simulink model "fec_ber_hw"  (R2020b)
settings: Solver=FixedStepDiscrete  StartTime=0.0  StopTime=T/2  RelTol=1e-3
values from neighbouring files (symbols this model uses):
  aximm_awgn_reset = 0    [setup.m]
  aximm_bit_count_reset = 0    [setup.m]
  aximm_bits = n_blocks * k    (= 3200)    [setup.m]
  aximm_ctrl_word_dec = 0    [setup.m]
  aximm_ctrl_word_enc = 0    [setup.m]
  aximm_enable = 1    [setup.m]
  aximm_length = k * n_blocks    (= 3200)    [setup.m]
  aximm_length_dec = n    (= 160)    [setup.m]
  aximm_length_enc = k    (= 80)    [setup.m]
  aximm_llr_mag_reset = 0    [setup.m]
  aximm_llr_scale = (1/noise_var) * llr_scale    (= 1000)    [setup.m]
  aximm_load_dec = 1    [setup.m]
  aximm_load_enc = 1    [setup.m]
  aximm_noise_std = sqrt(noise_var)    [setup.m]
  aximm_reset = 0    [setup.m]
  d = sqrt(-2*log([0:1/4095:1]))    [setup.m]
  fs = 160e6    (= 160000000)    [setup.m]
  llr_scale = 7.75/7.75    (= 1)    [setup.m]
libraries: simulink x450, hdlsllib x190, commseqgen3 x20, dspsigops x17, lib_rfsoc_fec x5, commblkcod2 x3
(part 22 of 22)

== system fec_ber_hw/Soft Demodulation/SSR Soft Demodulation Lane 1/Soft Demodulation 7/Subsystem1/get_min1 ==
  a : Inport
  b : Inport  Port=2
  Compare To Zero : simulink/Logic and Bit Operations/Compare To Zero  relop=<=  OutDataTypeStr=boolean
  Multiport Switch2 : MultiPortSwitch  DataPortOrder=Zero-based contiguous  Inputs=2  zeroidx=on
  Subtract18 : Sum  Inputs=+-  OutDataTypeStr=fixdt(1,(w+1)*2+2,f*2)  SaturateOnIntegerOverflow=on
  min : Outport
  wires:
  Subtract18/1 -> Compare To Zero/1
  b/1 -> Subtract18/2, Multiport Switch2/2
  a/1 -> Multiport Switch2/3, Subtract18/1
  Multiport Switch2/1 -> min/1
  Compare To Zero/1 -> Multiport Switch2/1

== system fec_ber_hw/Soft Demodulation/SSR Soft Demodulation Lane 1/Soft Demodulation 7/Subsystem1/get_min2 ==
  a : Inport
  b : Inport  Port=2
  Compare To Zero : simulink/Logic and Bit Operations/Compare To Zero  relop=<=  OutDataTypeStr=boolean
  Multiport Switch2 : MultiPortSwitch  DataPortOrder=Zero-based contiguous  Inputs=2  zeroidx=on
  Subtract18 : Sum  Inputs=+-  OutDataTypeStr=fixdt(1,(w+1)*2+2,f*2)  SaturateOnIntegerOverflow=on
  min : Outport
  wires:
  Compare To Zero/1 -> Multiport Switch2/1
  Multiport Switch2/1 -> min/1
  a/1 -> Subtract18/1, Multiport Switch2/3
  b/1 -> Multiport Switch2/2, Subtract18/2
  Subtract18/1 -> Compare To Zero/1

== system fec_ber_hw/Soft Demodulation/SSR Soft Demodulation Lane 1/Soft Demodulation 7/Subsystem1/get_min3 ==
  a : Inport
  b : Inport  Port=2
  Compare To Zero : simulink/Logic and Bit Operations/Compare To Zero  relop=<=  OutDataTypeStr=boolean
  Multiport Switch2 : MultiPortSwitch  DataPortOrder=Zero-based contiguous  Inputs=2  zeroidx=on
  Subtract18 : Sum  Inputs=+-  OutDataTypeStr=fixdt(1,(w+1)*2+2,f*2)  SaturateOnIntegerOverflow=on
  min : Outport
  wires:
  Subtract18/1 -> Compare To Zero/1
  b/1 -> Subtract18/2, Multiport Switch2/2
  a/1 -> Multiport Switch2/3, Subtract18/1
  Multiport Switch2/1 -> min/1
  Compare To Zero/1 -> Multiport Switch2/1

== system fec_ber_hw/Soft Demodulation/SSR Soft Demodulation Lane 1/Soft Demodulation 7/Subsystem1/get_min4 ==
  a : Inport
  b : Inport  Port=2
  Compare To Zero : simulink/Logic and Bit Operations/Compare To Zero  relop=<=  OutDataTypeStr=boolean
  Multiport Switch2 : MultiPortSwitch  DataPortOrder=Zero-based contiguous  Inputs=2  zeroidx=on
  Subtract18 : Sum  Inputs=+-  OutDataTypeStr=fixdt(1,(w+1)*2+2,f*2)  SaturateOnIntegerOverflow=on
  min : Outport
  wires:
  Compare To Zero/1 -> Multiport Switch2/1
  Multiport Switch2/1 -> min/1
  a/1 -> Subtract18/1, Multiport Switch2/3
  b/1 -> Multiport Switch2/2, Subtract18/2
  Subtract18/1 -> Compare To Zero/1

== system fec_ber_hw/Soft Demodulation/SSR Soft Demodulation Lane 1/Soft Demodulation 7/Subsystem1/get_min5 ==
  a : Inport
  b : Inport  Port=2
  Compare To Zero : simulink/Logic and Bit Operations/Compare To Zero  relop=<=  OutDataTypeStr=boolean
  Multiport Switch2 : MultiPortSwitch  DataPortOrder=Zero-based contiguous  Inputs=2  zeroidx=on
  Subtract18 : Sum  Inputs=+-  OutDataTypeStr=fixdt(1,(w+1)*2+2,f*2)  SaturateOnIntegerOverflow=on
  min : Outport
  wires:
  Subtract18/1 -> Compare To Zero/1
  b/1 -> Subtract18/2, Multiport Switch2/2
  a/1 -> Multiport Switch2/3, Subtract18/1
  Multiport Switch2/1 -> min/1
  Compare To Zero/1 -> Multiport Switch2/1

== system fec_ber_hw/Soft Demodulation/SSR Soft Demodulation Lane 1/Soft Demodulation 7/Subsystem1/get_min6 ==
  a : Inport
  b : Inport  Port=2
  Compare To Zero : simulink/Logic and Bit Operations/Compare To Zero  relop=<=  OutDataTypeStr=boolean
  Multiport Switch2 : MultiPortSwitch  DataPortOrder=Zero-based contiguous  Inputs=2  zeroidx=on
  Subtract18 : Sum  Inputs=+-  OutDataTypeStr=fixdt(1,(w+1)*2+2,f*2)  SaturateOnIntegerOverflow=on
  min : Outport
  wires:
  Compare To Zero/1 -> Multiport Switch2/1
  Multiport Switch2/1 -> min/1
  a/1 -> Subtract18/1, Multiport Switch2/3
  b/1 -> Multiport Switch2/2, Subtract18/2
  Subtract18/1 -> Compare To Zero/1

== system fec_ber_hw/Soft Demodulation/SSR Soft Demodulation Lane 1/Soft Demodulation 7/Subsystem1/get_min7 ==
  a : Inport
  b : Inport  Port=2
  Compare To Zero : simulink/Logic and Bit Operations/Compare To Zero  relop=<=  OutDataTypeStr=boolean
  Multiport Switch2 : MultiPortSwitch  DataPortOrder=Zero-based contiguous  Inputs=2  zeroidx=on
  Subtract18 : Sum  Inputs=+-  OutDataTypeStr=fixdt(1,(w+1)*2+2,f*2)  SaturateOnIntegerOverflow=on
  min : Outport
  wires:
  Compare To Zero/1 -> Multiport Switch2/1
  Multiport Switch2/1 -> min/1
  a/1 -> Subtract18/1, Multiport Switch2/3
  b/1 -> Multiport Switch2/2, Subtract18/2
  Subtract18/1 -> Compare To Zero/1

== system fec_ber_hw/Soft Demodulation/SSR Soft Demodulation Lane 1/Soft Demodulation 7/Subsystem2/get_min1 ==
  a : Inport
  b : Inport  Port=2
  Compare To Zero : simulink/Logic and Bit Operations/Compare To Zero  relop=<=  OutDataTypeStr=boolean
  Multiport Switch2 : MultiPortSwitch  DataPortOrder=Zero-based contiguous  Inputs=2  zeroidx=on
  Subtract18 : Sum  Inputs=+-  OutDataTypeStr=fixdt(1,(w+1)*2+2,f*2)  SaturateOnIntegerOverflow=on
  min : Outport
  wires:
  Subtract18/1 -> Compare To Zero/1
  b/1 -> Subtract18/2, Multiport Switch2/2
  a/1 -> Multiport Switch2/3, Subtract18/1
  Multiport Switch2/1 -> min/1
  Compare To Zero/1 -> Multiport Switch2/1

== system fec_ber_hw/Soft Demodulation/SSR Soft Demodulation Lane 1/Soft Demodulation 7/Subsystem2/get_min2 ==
  a : Inport
  b : Inport  Port=2
  Compare To Zero : simulink/Logic and Bit Operations/Compare To Zero  relop=<=  OutDataTypeStr=boolean
  Multiport Switch2 : MultiPortSwitch  DataPortOrder=Zero-based contiguous  Inputs=2  zeroidx=on
  Subtract18 : Sum  Inputs=+-  OutDataTypeStr=fixdt(1,(w+1)*2+2,f*2)  SaturateOnIntegerOverflow=on
  min : Outport
  wires:
  Compare To Zero/1 -> Multiport Switch2/1
  Multiport Switch2/1 -> min/1
  a/1 -> Subtract18/1, Multiport Switch2/3
  b/1 -> Multiport Switch2/2, Subtract18/2
  Subtract18/1 -> Compare To Zero/1

== system fec_ber_hw/Soft Demodulation/SSR Soft Demodulation Lane 1/Soft Demodulation 7/Subsystem2/get_min3 ==
  a : Inport
  b : Inport  Port=2
  Compare To Zero : simulink/Logic and Bit Operations/Compare To Zero  relop=<=  OutDataTypeStr=boolean
  Multiport Switch2 : MultiPortSwitch  DataPortOrder=Zero-based contiguous  Inputs=2  zeroidx=on
  Subtract18 : Sum  Inputs=+-  OutDataTypeStr=fixdt(1,(w+1)*2+2,f*2)  SaturateOnIntegerOverflow=on
  min : Outport
  wires:
  Subtract18/1 -> Compare To Zero/1
  b/1 -> Subtract18/2, Multiport Switch2/2
  a/1 -> Multiport Switch2/3, Subtract18/1
  Multiport Switch2/1 -> min/1
  Compare To Zero/1 -> Multiport Switch2/1

== system fec_ber_hw/Soft Demodulation/SSR Soft Demodulation Lane 1/Soft Demodulation 7/Subsystem2/get_min4 ==
  a : Inport
  b : Inport  Port=2
  Compare To Zero : simulink/Logic and Bit Operations/Compare To Zero  relop=<=  OutDataTypeStr=boolean
  Multiport Switch2 : MultiPortSwitch  DataPortOrder=Zero-based contiguous  Inputs=2  zeroidx=on
  Subtract18 : Sum  Inputs=+-  OutDataTypeStr=fixdt(1,(w+1)*2+2,f*2)  SaturateOnIntegerOverflow=on
  min : Outport
  wires:
  Compare To Zero/1 -> Multiport Switch2/1
  Multiport Switch2/1 -> min/1
  a/1 -> Subtract18/1, Multiport Switch2/3
  b/1 -> Multiport Switch2/2, Subtract18/2
  Subtract18/1 -> Compare To Zero/1

== system fec_ber_hw/Soft Demodulation/SSR Soft Demodulation Lane 1/Soft Demodulation 7/Subsystem2/get_min5 ==
  a : Inport
  b : Inport  Port=2
  Compare To Zero : simulink/Logic and Bit Operations/Compare To Zero  relop=<=  OutDataTypeStr=boolean
  Multiport Switch2 : MultiPortSwitch  DataPortOrder=Zero-based contiguous  Inputs=2  zeroidx=on
  Subtract18 : Sum  Inputs=+-  OutDataTypeStr=fixdt(1,(w+1)*2+2,f*2)  SaturateOnIntegerOverflow=on
  min : Outport
  wires:
  Subtract18/1 -> Compare To Zero/1
  b/1 -> Subtract18/2, Multiport Switch2/2
  a/1 -> Multiport Switch2/3, Subtract18/1
  Multiport Switch2/1 -> min/1
  Compare To Zero/1 -> Multiport Switch2/1

== system fec_ber_hw/Soft Demodulation/SSR Soft Demodulation Lane 1/Soft Demodulation 7/Subsystem2/get_min6 ==
  a : Inport
  b : Inport  Port=2
  Compare To Zero : simulink/Logic and Bit Operations/Compare To Zero  relop=<=  OutDataTypeStr=boolean
  Multiport Switch2 : MultiPortSwitch  DataPortOrder=Zero-based contiguous  Inputs=2  zeroidx=on
  Subtract18 : Sum  Inputs=+-  OutDataTypeStr=fixdt(1,(w+1)*2+2,f*2)  SaturateOnIntegerOverflow=on
  min : Outport
  wires:
  Compare To Zero/1 -> Multiport Switch2/1
  Multiport Switch2/1 -> min/1
  a/1 -> Subtract18/1, Multiport Switch2/3
  b/1 -> Multiport Switch2/2, Subtract18/2
  Subtract18/1 -> Compare To Zero/1

== system fec_ber_hw/Soft Demodulation/SSR Soft Demodulation Lane 1/Soft Demodulation 7/Subsystem2/get_min7 ==
  a : Inport
  b : Inport  Port=2
  Compare To Zero : simulink/Logic and Bit Operations/Compare To Zero  relop=<=  OutDataTypeStr=boolean
  Multiport Switch2 : MultiPortSwitch  DataPortOrder=Zero-based contiguous  Inputs=2  zeroidx=on
  Subtract18 : Sum  Inputs=+-  OutDataTypeStr=fixdt(1,(w+1)*2+2,f*2)  SaturateOnIntegerOverflow=on
  min : Outport
  wires:
  Compare To Zero/1 -> Multiport Switch2/1
  Multiport Switch2/1 -> min/1
  a/1 -> Subtract18/1, Multiport Switch2/3
  b/1 -> Multiport Switch2/2, Subtract18/2
  Subtract18/1 -> Compare To Zero/1

== system fec_ber_hw/Soft Demodulation/SSR Soft Demodulation Lane 1/Soft Demodulation 8/Subsystem1/get_min1 ==
  a : Inport
  b : Inport  Port=2
  Compare To Zero : simulink/Logic and Bit Operations/Compare To Zero  relop=<=  OutDataTypeStr=boolean
  Multiport Switch2 : MultiPortSwitch  DataPortOrder=Zero-based contiguous  Inputs=2  zeroidx=on
  Subtract18 : Sum  Inputs=+-  OutDataTypeStr=fixdt(1,(w+1)*2+2,f*2)  SaturateOnIntegerOverflow=on
  min : Outport
  wires:
  Subtract18/1 -> Compare To Zero/1
  b/1 -> Subtract18/2, Multiport Switch2/2
  a/1 -> Multiport Switch2/3, Subtract18/1
  Multiport Switch2/1 -> min/1
  Compare To Zero/1 -> Multiport Switch2/1

== system fec_ber_hw/Soft Demodulation/SSR Soft Demodulation Lane 1/Soft Demodulation 8/Subsystem1/get_min2 ==
  a : Inport
  b : Inport  Port=2
  Compare To Zero : simulink/Logic and Bit Operations/Compare To Zero  relop=<=  OutDataTypeStr=boolean
  Multiport Switch2 : MultiPortSwitch  DataPortOrder=Zero-based contiguous  Inputs=2  zeroidx=on
  Subtract18 : Sum  Inputs=+-  OutDataTypeStr=fixdt(1,(w+1)*2+2,f*2)  SaturateOnIntegerOverflow=on
  min : Outport
  wires:
  Compare To Zero/1 -> Multiport Switch2/1
  Multiport Switch2/1 -> min/1
  a/1 -> Subtract18/1, Multiport Switch2/3
  b/1 -> Multiport Switch2/2, Subtract18/2
  Subtract18/1 -> Compare To Zero/1

== system fec_ber_hw/Soft Demodulation/SSR Soft Demodulation Lane 1/Soft Demodulation 8/Subsystem1/get_min3 ==
  a : Inport
  b : Inport  Port=2
  Compare To Zero : simulink/Logic and Bit Operations/Compare To Zero  relop=<=  OutDataTypeStr=boolean
  Multiport Switch2 : MultiPortSwitch  DataPortOrder=Zero-based contiguous  Inputs=2  zeroidx=on
  Subtract18 : Sum  Inputs=+-  OutDataTypeStr=fixdt(1,(w+1)*2+2,f*2)  SaturateOnIntegerOverflow=on
  min : Outport
  wires:
  Subtract18/1 -> Compare To Zero/1
  b/1 -> Subtract18/2, Multiport Switch2/2
  a/1 -> Multiport Switch2/3, Subtract18/1
  Multiport Switch2/1 -> min/1
  Compare To Zero/1 -> Multiport Switch2/1

== system fec_ber_hw/Soft Demodulation/SSR Soft Demodulation Lane 1/Soft Demodulation 8/Subsystem1/get_min4 ==
  a : Inport
  b : Inport  Port=2
  Compare To Zero : simulink/Logic and Bit Operations/Compare To Zero  relop=<=  OutDataTypeStr=boolean
  Multiport Switch2 : MultiPortSwitch  DataPortOrder=Zero-based contiguous  Inputs=2  zeroidx=on
  Subtract18 : Sum  Inputs=+-  OutDataTypeStr=fixdt(1,(w+1)*2+2,f*2)  SaturateOnIntegerOverflow=on
  min : Outport
  wires:
  Compare To Zero/1 -> Multiport Switch2/1
  Multiport Switch2/1 -> min/1
  a/1 -> Subtract18/1, Multiport Switch2/3
  b/1 -> Multiport Switch2/2, Subtract18/2
  Subtract18/1 -> Compare To Zero/1

== system fec_ber_hw/Soft Demodulation/SSR Soft Demodulation Lane 1/Soft Demodulation 8/Subsystem1/get_min5 ==
  a : Inport
  b : Inport  Port=2
  Compare To Zero : simulink/Logic and Bit Operations/Compare To Zero  relop=<=  OutDataTypeStr=boolean
  Multiport Switch2 : MultiPortSwitch  DataPortOrder=Zero-based contiguous  Inputs=2  zeroidx=on
  Subtract18 : Sum  Inputs=+-  OutDataTypeStr=fixdt(1,(w+1)*2+2,f*2)  SaturateOnIntegerOverflow=on
  min : Outport
  wires:
  Subtract18/1 -> Compare To Zero/1
  b/1 -> Subtract18/2, Multiport Switch2/2
  a/1 -> Multiport Switch2/3, Subtract18/1
  Multiport Switch2/1 -> min/1
  Compare To Zero/1 -> Multiport Switch2/1

== system fec_ber_hw/Soft Demodulation/SSR Soft Demodulation Lane 1/Soft Demodulation 8/Subsystem1/get_min6 ==
  a : Inport
  b : Inport  Port=2
  Compare To Zero : simulink/Logic and Bit Operations/Compare To Zero  relop=<=  OutDataTypeStr=boolean
  Multiport Switch2 : MultiPortSwitch  DataPortOrder=Zero-based contiguous  Inputs=2  zeroidx=on
  Subtract18 : Sum  Inputs=+-  OutDataTypeStr=fixdt(1,(w+1)*2+2,f*2)  SaturateOnIntegerOverflow=on
  min : Outport
  wires:
  Compare To Zero/1 -> Multiport Switch2/1
  Multiport Switch2/1 -> min/1
  a/1 -> Subtract18/1, Multiport Switch2/3
  b/1 -> Multiport Switch2/2, Subtract18/2
  Subtract18/1 -> Compare To Zero/1

== system fec_ber_hw/Soft Demodulation/SSR Soft Demodulation Lane 1/Soft Demodulation 8/Subsystem1/get_min7 ==
  a : Inport
  b : Inport  Port=2
  Compare To Zero : simulink/Logic and Bit Operations/Compare To Zero  relop=<=  OutDataTypeStr=boolean
  Multiport Switch2 : MultiPortSwitch  DataPortOrder=Zero-based contiguous  Inputs=2  zeroidx=on
  Subtract18 : Sum  Inputs=+-  OutDataTypeStr=fixdt(1,(w+1)*2+2,f*2)  SaturateOnIntegerOverflow=on
  min : Outport
  wires:
  Compare To Zero/1 -> Multiport Switch2/1
  Multiport Switch2/1 -> min/1
  a/1 -> Subtract18/1, Multiport Switch2/3
  b/1 -> Multiport Switch2/2, Subtract18/2
  Subtract18/1 -> Compare To Zero/1

== system fec_ber_hw/Soft Demodulation/SSR Soft Demodulation Lane 1/Soft Demodulation 8/Subsystem2/get_min1 ==
  a : Inport
  b : Inport  Port=2
  Compare To Zero : simulink/Logic and Bit Operations/Compare To Zero  relop=<=  OutDataTypeStr=boolean
  Multiport Switch2 : MultiPortSwitch  DataPortOrder=Zero-based contiguous  Inputs=2  zeroidx=on
  Subtract18 : Sum  Inputs=+-  OutDataTypeStr=fixdt(1,(w+1)*2+2,f*2)  SaturateOnIntegerOverflow=on
  min : Outport
  wires:
  Subtract18/1 -> Compare To Zero/1
  b/1 -> Subtract18/2, Multiport Switch2/2
  a/1 -> Multiport Switch2/3, Subtract18/1
  Multiport Switch2/1 -> min/1
  Compare To Zero/1 -> Multiport Switch2/1

== system fec_ber_hw/Soft Demodulation/SSR Soft Demodulation Lane 1/Soft Demodulation 8/Subsystem2/get_min2 ==
  a : Inport
  b : Inport  Port=2
  Compare To Zero : simulink/Logic and Bit Operations/Compare To Zero  relop=<=  OutDataTypeStr=boolean
  Multiport Switch2 : MultiPortSwitch  DataPortOrder=Zero-based contiguous  Inputs=2  zeroidx=on
  Subtract18 : Sum  Inputs=+-  OutDataTypeStr=fixdt(1,(w+1)*2+2,f*2)  SaturateOnIntegerOverflow=on
  min : Outport
  wires:
  Compare To Zero/1 -> Multiport Switch2/1
  Multiport Switch2/1 -> min/1
  a/1 -> Subtract18/1, Multiport Switch2/3
  b/1 -> Multiport Switch2/2, Subtract18/2
  Subtract18/1 -> Compare To Zero/1

== system fec_ber_hw/Soft Demodulation/SSR Soft Demodulation Lane 1/Soft Demodulation 8/Subsystem2/get_min3 ==
  a : Inport
  b : Inport  Port=2
  Compare To Zero : simulink/Logic and Bit Operations/Compare To Zero  relop=<=  OutDataTypeStr=boolean
  Multiport Switch2 : MultiPortSwitch  DataPortOrder=Zero-based contiguous  Inputs=2  zeroidx=on
  Subtract18 : Sum  Inputs=+-  OutDataTypeStr=fixdt(1,(w+1)*2+2,f*2)  SaturateOnIntegerOverflow=on
  min : Outport
  wires:
  Subtract18/1 -> Compare To Zero/1
  b/1 -> Subtract18/2, Multiport Switch2/2
  a/1 -> Multiport Switch2/3, Subtract18/1
  Multiport Switch2/1 -> min/1
  Compare To Zero/1 -> Multiport Switch2/1

== system fec_ber_hw/Soft Demodulation/SSR Soft Demodulation Lane 1/Soft Demodulation 8/Subsystem2/get_min4 ==
  a : Inport
  b : Inport  Port=2
  Compare To Zero : simulink/Logic and Bit Operations/Compare To Zero  relop=<=  OutDataTypeStr=boolean
  Multiport Switch2 : MultiPortSwitch  DataPortOrder=Zero-based contiguous  Inputs=2  zeroidx=on
  Subtract18 : Sum  Inputs=+-  OutDataTypeStr=fixdt(1,(w+1)*2+2,f*2)  SaturateOnIntegerOverflow=on
  min : Outport
  wires:
  Compare To Zero/1 -> Multiport Switch2/1
  Multiport Switch2/1 -> min/1
  a/1 -> Subtract18/1, Multiport Switch2/3
  b/1 -> Multiport Switch2/2, Subtract18/2
  Subtract18/1 -> Compare To Zero/1

== system fec_ber_hw/Soft Demodulation/SSR Soft Demodulation Lane 1/Soft Demodulation 8/Subsystem2/get_min5 ==
  a : Inport
  b : Inport  Port=2
  Compare To Zero : simulink/Logic and Bit Operations/Compare To Zero  relop=<=  OutDataTypeStr=boolean
  Multiport Switch2 : MultiPortSwitch  DataPortOrder=Zero-based contiguous  Inputs=2  zeroidx=on
  Subtract18 : Sum  Inputs=+-  OutDataTypeStr=fixdt(1,(w+1)*2+2,f*2)  SaturateOnIntegerOverflow=on
  min : Outport
  wires:
  Subtract18/1 -> Compare To Zero/1
  b/1 -> Subtract18/2, Multiport Switch2/2
  a/1 -> Multiport Switch2/3, Subtract18/1
  Multiport Switch2/1 -> min/1
  Compare To Zero/1 -> Multiport Switch2/1

== system fec_ber_hw/Soft Demodulation/SSR Soft Demodulation Lane 1/Soft Demodulation 8/Subsystem2/get_min6 ==
  a : Inport
  b : Inport  Port=2
  Compare To Zero : simulink/Logic and Bit Operations/Compare To Zero  relop=<=  OutDataTypeStr=boolean
  Multiport Switch2 : MultiPortSwitch  DataPortOrder=Zero-based contiguous  Inputs=2  zeroidx=on
  Subtract18 : Sum  Inputs=+-  OutDataTypeStr=fixdt(1,(w+1)*2+2,f*2)  SaturateOnIntegerOverflow=on
  min : Outport
  wires:
  Compare To Zero/1 -> Multiport Switch2/1
  Multiport Switch2/1 -> min/1
  a/1 -> Subtract18/1, Multiport Switch2/3
  b/1 -> Multiport Switch2/2, Subtract18/2
  Subtract18/1 -> Compare To Zero/1

== system fec_ber_hw/Soft Demodulation/SSR Soft Demodulation Lane 1/Soft Demodulation 8/Subsystem2/get_min7 ==
  a : Inport
  b : Inport  Port=2
  Compare To Zero : simulink/Logic and Bit Operations/Compare To Zero  relop=<=  OutDataTypeStr=boolean
  Multiport Switch2 : MultiPortSwitch  DataPortOrder=Zero-based contiguous  Inputs=2  zeroidx=on
  Subtract18 : Sum  Inputs=+-  OutDataTypeStr=fixdt(1,(w+1)*2+2,f*2)  SaturateOnIntegerOverflow=on
  min : Outport
  wires:
  Compare To Zero/1 -> Multiport Switch2/1
  Multiport Switch2/1 -> min/1
  a/1 -> Subtract18/1, Multiport Switch2/3
  b/1 -> Multiport Switch2/2, Subtract18/2
  Subtract18/1 -> Compare To Zero/1

== system fec_ber_hw/Soft Demodulation/SSR Soft Demodulation Lane 1/Soft Demodulation 9/Subsystem1/get_min1 ==
  a : Inport
  b : Inport  Port=2
  Compare To Zero : simulink/Logic and Bit Operations/Compare To Zero  relop=<=  OutDataTypeStr=boolean
  Multiport Switch2 : MultiPortSwitch  DataPortOrder=Zero-based contiguous  Inputs=2  zeroidx=on
  Subtract18 : Sum  Inputs=+-  OutDataTypeStr=fixdt(1,(w+1)*2+2,f*2)  SaturateOnIntegerOverflow=on
  min : Outport
  wires:
  Subtract18/1 -> Compare To Zero/1
  b/1 -> Subtract18/2, Multiport Switch2/2
  a/1 -> Multiport Switch2/3, Subtract18/1
  Multiport Switch2/1 -> min/1
  Compare To Zero/1 -> Multiport Switch2/1

== system fec_ber_hw/Soft Demodulation/SSR Soft Demodulation Lane 1/Soft Demodulation 9/Subsystem1/get_min2 ==
  a : Inport
  b : Inport  Port=2
  Compare To Zero : simulink/Logic and Bit Operations/Compare To Zero  relop=<=  OutDataTypeStr=boolean
  Multiport Switch2 : MultiPortSwitch  DataPortOrder=Zero-based contiguous  Inputs=2  zeroidx=on
  Subtract18 : Sum  Inputs=+-  OutDataTypeStr=fixdt(1,(w+1)*2+2,f*2)  SaturateOnIntegerOverflow=on
  min : Outport
  wires:
  Compare To Zero/1 -> Multiport Switch2/1
  Multiport Switch2/1 -> min/1
  a/1 -> Subtract18/1, Multiport Switch2/3
  b/1 -> Multiport Switch2/2, Subtract18/2
  Subtract18/1 -> Compare To Zero/1

== system fec_ber_hw/Soft Demodulation/SSR Soft Demodulation Lane 1/Soft Demodulation 9/Subsystem1/get_min3 ==
  a : Inport
  b : Inport  Port=2
  Compare To Zero : simulink/Logic and Bit Operations/Compare To Zero  relop=<=  OutDataTypeStr=boolean
  Multiport Switch2 : MultiPortSwitch  DataPortOrder=Zero-based contiguous  Inputs=2  zeroidx=on
  Subtract18 : Sum  Inputs=+-  OutDataTypeStr=fixdt(1,(w+1)*2+2,f*2)  SaturateOnIntegerOverflow=on
  min : Outport
  wires:
  Subtract18/1 -> Compare To Zero/1
  b/1 -> Subtract18/2, Multiport Switch2/2
  a/1 -> Multiport Switch2/3, Subtract18/1
  Multiport Switch2/1 -> min/1
  Compare To Zero/1 -> Multiport Switch2/1

== system fec_ber_hw/Soft Demodulation/SSR Soft Demodulation Lane 1/Soft Demodulation 9/Subsystem1/get_min4 ==
  a : Inport
  b : Inport  Port=2
  Compare To Zero : simulink/Logic and Bit Operations/Compare To Zero  relop=<=  OutDataTypeStr=boolean
  Multiport Switch2 : MultiPortSwitch  DataPortOrder=Zero-based contiguous  Inputs=2  zeroidx=on
  Subtract18 : Sum  Inputs=+-  OutDataTypeStr=fixdt(1,(w+1)*2+2,f*2)  SaturateOnIntegerOverflow=on
  min : Outport
  wires:
  Compare To Zero/1 -> Multiport Switch2/1
  Multiport Switch2/1 -> min/1
  a/1 -> Subtract18/1, Multiport Switch2/3
  b/1 -> Multiport Switch2/2, Subtract18/2
  Subtract18/1 -> Compare To Zero/1

== system fec_ber_hw/Soft Demodulation/SSR Soft Demodulation Lane 1/Soft Demodulation 9/Subsystem1/get_min5 ==
  a : Inport
  b : Inport  Port=2
  Compare To Zero : simulink/Logic and Bit Operations/Compare To Zero  relop=<=  OutDataTypeStr=boolean
  Multiport Switch2 : MultiPortSwitch  DataPortOrder=Zero-based contiguous  Inputs=2  zeroidx=on
  Subtract18 : Sum  Inputs=+-  OutDataTypeStr=fixdt(1,(w+1)*2+2,f*2)  SaturateOnIntegerOverflow=on
  min : Outport
  wires:
  Subtract18/1 -> Compare To Zero/1
  b/1 -> Subtract18/2, Multiport Switch2/2
  a/1 -> Multiport Switch2/3, Subtract18/1
  Multiport Switch2/1 -> min/1
  Compare To Zero/1 -> Multiport Switch2/1

== system fec_ber_hw/Soft Demodulation/SSR Soft Demodulation Lane 1/Soft Demodulation 9/Subsystem1/get_min6 ==
  a : Inport
  b : Inport  Port=2
  Compare To Zero : simulink/Logic and Bit Operations/Compare To Zero  relop=<=  OutDataTypeStr=boolean
  Multiport Switch2 : MultiPortSwitch  DataPortOrder=Zero-based contiguous  Inputs=2  zeroidx=on
  Subtract18 : Sum  Inputs=+-  OutDataTypeStr=fixdt(1,(w+1)*2+2,f*2)  SaturateOnIntegerOverflow=on
  min : Outport
  wires:
  Compare To Zero/1 -> Multiport Switch2/1
  Multiport Switch2/1 -> min/1
  a/1 -> Subtract18/1, Multiport Switch2/3
  b/1 -> Multiport Switch2/2, Subtract18/2
  Subtract18/1 -> Compare To Zero/1

== system fec_ber_hw/Soft Demodulation/SSR Soft Demodulation Lane 1/Soft Demodulation 9/Subsystem1/get_min7 ==
  a : Inport
  b : Inport  Port=2
  Compare To Zero : simulink/Logic and Bit Operations/Compare To Zero  relop=<=  OutDataTypeStr=boolean
  Multiport Switch2 : MultiPortSwitch  DataPortOrder=Zero-based contiguous  Inputs=2  zeroidx=on
  Subtract18 : Sum  Inputs=+-  OutDataTypeStr=fixdt(1,(w+1)*2+2,f*2)  SaturateOnIntegerOverflow=on
  min : Outport
  wires:
  Compare To Zero/1 -> Multiport Switch2/1
  Multiport Switch2/1 -> min/1
  a/1 -> Subtract18/1, Multiport Switch2/3
  b/1 -> Multiport Switch2/2, Subtract18/2
  Subtract18/1 -> Compare To Zero/1

== system fec_ber_hw/Soft Demodulation/SSR Soft Demodulation Lane 1/Soft Demodulation 9/Subsystem2/get_min1 ==
  a : Inport
  b : Inport  Port=2
  Compare To Zero : simulink/Logic and Bit Operations/Compare To Zero  relop=<=  OutDataTypeStr=boolean
  Multiport Switch2 : MultiPortSwitch  DataPortOrder=Zero-based contiguous  Inputs=2  zeroidx=on
  Subtract18 : Sum  Inputs=+-  OutDataTypeStr=fixdt(1,(w+1)*2+2,f*2)  SaturateOnIntegerOverflow=on
  min : Outport
  wires:
  Subtract18/1 -> Compare To Zero/1
  b/1 -> Subtract18/2, Multiport Switch2/2
  a/1 -> Multiport Switch2/3, Subtract18/1
  Multiport Switch2/1 -> min/1
  Compare To Zero/1 -> Multiport Switch2/1

== system fec_ber_hw/Soft Demodulation/SSR Soft Demodulation Lane 1/Soft Demodulation 9/Subsystem2/get_min2 ==
  a : Inport
  b : Inport  Port=2
  Compare To Zero : simulink/Logic and Bit Operations/Compare To Zero  relop=<=  OutDataTypeStr=boolean
  Multiport Switch2 : MultiPortSwitch  DataPortOrder=Zero-based contiguous  Inputs=2  zeroidx=on
  Subtract18 : Sum  Inputs=+-  OutDataTypeStr=fixdt(1,(w+1)*2+2,f*2)  SaturateOnIntegerOverflow=on
  min : Outport
  wires:
  Compare To Zero/1 -> Multiport Switch2/1
  Multiport Switch2/1 -> min/1
  a/1 -> Subtract18/1, Multiport Switch2/3
  b/1 -> Multiport Switch2/2, Subtract18/2
  Subtract18/1 -> Compare To Zero/1

== system fec_ber_hw/Soft Demodulation/SSR Soft Demodulation Lane 1/Soft Demodulation 9/Subsystem2/get_min3 ==
  a : Inport
  b : Inport  Port=2
  Compare To Zero : simulink/Logic and Bit Operations/Compare To Zero  relop=<=  OutDataTypeStr=boolean
  Multiport Switch2 : MultiPortSwitch  DataPortOrder=Zero-based contiguous  Inputs=2  zeroidx=on
  Subtract18 : Sum  Inputs=+-  OutDataTypeStr=fixdt(1,(w+1)*2+2,f*2)  SaturateOnIntegerOverflow=on
  min : Outport
  wires:
  Subtract18/1 -> Compare To Zero/1
  b/1 -> Subtract18/2, Multiport Switch2/2
  a/1 -> Multiport Switch2/3, Subtract18/1
  Multiport Switch2/1 -> min/1
  Compare To Zero/1 -> Multiport Switch2/1

== system fec_ber_hw/Soft Demodulation/SSR Soft Demodulation Lane 1/Soft Demodulation 9/Subsystem2/get_min4 ==
  a : Inport
  b : Inport  Port=2
  Compare To Zero : simulink/Logic and Bit Operations/Compare To Zero  relop=<=  OutDataTypeStr=boolean
  Multiport Switch2 : MultiPortSwitch  DataPortOrder=Zero-based contiguous  Inputs=2  zeroidx=on
  Subtract18 : Sum  Inputs=+-  OutDataTypeStr=fixdt(1,(w+1)*2+2,f*2)  SaturateOnIntegerOverflow=on
  min : Outport
  wires:
  Compare To Zero/1 -> Multiport Switch2/1
  Multiport Switch2/1 -> min/1
  a/1 -> Subtract18/1, Multiport Switch2/3
  b/1 -> Multiport Switch2/2, Subtract18/2
  Subtract18/1 -> Compare To Zero/1

== system fec_ber_hw/Soft Demodulation/SSR Soft Demodulation Lane 1/Soft Demodulation 9/Subsystem2/get_min5 ==
  a : Inport
  b : Inport  Port=2
  Compare To Zero : simulink/Logic and Bit Operations/Compare To Zero  relop=<=  OutDataTypeStr=boolean
  Multiport Switch2 : MultiPortSwitch  DataPortOrder=Zero-based contiguous  Inputs=2  zeroidx=on
  Subtract18 : Sum  Inputs=+-  OutDataTypeStr=fixdt(1,(w+1)*2+2,f*2)  SaturateOnIntegerOverflow=on
  min : Outport
  wires:
  Subtract18/1 -> Compare To Zero/1
  b/1 -> Subtract18/2, Multiport Switch2/2
  a/1 -> Multiport Switch2/3, Subtract18/1
  Multiport Switch2/1 -> min/1
  Compare To Zero/1 -> Multiport Switch2/1

== system fec_ber_hw/Soft Demodulation/SSR Soft Demodulation Lane 1/Soft Demodulation 9/Subsystem2/get_min6 ==
  a : Inport
  b : Inport  Port=2
  Compare To Zero : simulink/Logic and Bit Operations/Compare To Zero  relop=<=  OutDataTypeStr=boolean
  Multiport Switch2 : MultiPortSwitch  DataPortOrder=Zero-based contiguous  Inputs=2  zeroidx=on
  Subtract18 : Sum  Inputs=+-  OutDataTypeStr=fixdt(1,(w+1)*2+2,f*2)  SaturateOnIntegerOverflow=on
  min : Outport
  wires:
  Compare To Zero/1 -> Multiport Switch2/1
  Multiport Switch2/1 -> min/1
  a/1 -> Subtract18/1, Multiport Switch2/3
  b/1 -> Multiport Switch2/2, Subtract18/2
  Subtract18/1 -> Compare To Zero/1

== system fec_ber_hw/Soft Demodulation/SSR Soft Demodulation Lane 1/Soft Demodulation 9/Subsystem2/get_min7 ==
  a : Inport
  b : Inport  Port=2
  Compare To Zero : simulink/Logic and Bit Operations/Compare To Zero  relop=<=  OutDataTypeStr=boolean
  Multiport Switch2 : MultiPortSwitch  DataPortOrder=Zero-based contiguous  Inputs=2  zeroidx=on
  Subtract18 : Sum  Inputs=+-  OutDataTypeStr=fixdt(1,(w+1)*2+2,f*2)  SaturateOnIntegerOverflow=on
  min : Outport
  wires:
  Compare To Zero/1 -> Multiport Switch2/1
  Multiport Switch2/1 -> min/1
  a/1 -> Subtract18/1, Multiport Switch2/3
  b/1 -> Multiport Switch2/2, Subtract18/2
  Subtract18/1 -> Compare To Zero/1

== matlab function fec_ber_hw/Decode/MATLAB Function1 ==
  data: valid input; frame input; uint8 output [0..80]; k parameter
function uint8 = fcn(valid, frame, k)

persistent f u count

if isempty(f)
    f = zeros(1,8);
    u = fi(0,0,8,0);
    count = 0;
end

if valid
    f = frame((1:8)+(8*count));
    u(:) = f(8)*2^7 ...
      + f(7)*2^6 ...
      + f(6)*2^5 ...
      + f(5)*2^4 ...
      + f(4)*2^3 ...
      + f(3)*2^2 ...
      + f(2)*2^1 ...
      + f(1)*2^0;
  count = count + 1;
end

if count >= 10
    count = 0;
end

uint8 = u;

== matlab function fec_ber_hw/Soft Demodulation/SSR Soft Demodulation Lane 0/Soft Demodulation 2/symmetric_saturation ==
  data: u input; y output
function y = symmetric_saturation(u)
    if u > 7.75
        y = fi(7.75, 1, 6, 2);
    elseif u < -7.75
        y = fi(-7.75, 1, 6, 2);
    else
        y = fi(u, 1, 6, 2);
    end

== matlab function fec_ber_hw/Soft Demodulation/SSR Soft Demodulation Lane 0/Soft Demodulation 3/symmetric_saturation ==
  data: u input; y output
function y = symmetric_saturation(u)
    if u > 7.75
        y = fi(7.75, 1, 6, 2);
    elseif u < -7.75
        y = fi(-7.75, 1, 6, 2);
    else
        y = fi(u, 1, 6, 2);
    end

== matlab function fec_ber_hw/Soft Demodulation/SSR Soft Demodulation Lane 0/Soft Demodulation 4/symmetric_saturation ==
  data: u input; y output
function y = symmetric_saturation(u)
    if u > 7.75
        y = fi(7.75, 1, 6, 2);
    elseif u < -7.75
        y = fi(-7.75, 1, 6, 2);
    else
        y = fi(u, 1, 6, 2);
    end

== matlab function fec_ber_hw/Soft Demodulation/SSR Soft Demodulation Lane 0/Soft Demodulation 5/symmetric_saturation ==
  data: u input; y output
function y = symmetric_saturation(u)
    if u > 7.75
        y = fi(7.75, 1, 6, 2);
    elseif u < -7.75
        y = fi(-7.75, 1, 6, 2);
    else
        y = fi(u, 1, 6, 2);
    end

== matlab function fec_ber_hw/Soft Demodulation/SSR Soft Demodulation Lane 0/Soft Demodulation 6/symmetric_saturation ==
  data: u input; y output
function y = symmetric_saturation(u)
    if u > 7.75
        y = fi(7.75, 1, 6, 2);
    elseif u < -7.75
        y = fi(-7.75, 1, 6, 2);
    else
        y = fi(u, 1, 6, 2);
    end

== matlab function fec_ber_hw/Soft Demodulation/SSR Soft Demodulation Lane 0/Soft Demodulation 7/symmetric_saturation ==
  data: u input; y output
function y = symmetric_saturation(u)
    if u > 7.75
        y = fi(7.75, 1, 6, 2);
    elseif u < -7.75
        y = fi(-7.75, 1, 6, 2);
    else
        y = fi(u, 1, 6, 2);
    end

== matlab function fec_ber_hw/Soft Demodulation/SSR Soft Demodulation Lane 0/Soft Demodulation 8/symmetric_saturation ==
  data: u input; y output
function y = symmetric_saturation(u)
    if u > 7.75
        y = fi(7.75, 1, 6, 2);
    elseif u < -7.75
        y = fi(-7.75, 1, 6, 2);
    else
        y = fi(u, 1, 6, 2);
    end

== matlab function fec_ber_hw/Soft Demodulation/SSR Soft Demodulation Lane 0/Soft Demodulation 9/symmetric_saturation ==
  data: u input; y output
function y = symmetric_saturation(u)
    if u > 7.75
        y = fi(7.75, 1, 6, 2);
    elseif u < -7.75
        y = fi(-7.75, 1, 6, 2);
    else
        y = fi(u, 1, 6, 2);
    end

== matlab function fec_ber_hw/Soft Demodulation/SSR Soft Demodulation Lane 0/Soft Demodulation 10/symmetric_saturation ==
  data: u input; y output
function y = symmetric_saturation(u)
    if u > 7.75
        y = fi(7.75, 1, 6, 2);
    elseif u < -7.75
        y = fi(-7.75, 1, 6, 2);
    else
        y = fi(u, 1, 6, 2);
    end

== matlab function fec_ber_hw/Soft Demodulation/SSR Soft Demodulation Lane 0/Soft Demodulation 11/symmetric_saturation ==
  data: u input; y output
function y = symmetric_saturation(u)
    if u > 7.75
        y = fi(7.75, 1, 6, 2);
    elseif u < -7.75
        y = fi(-7.75, 1, 6, 2);
    else
        y = fi(u, 1, 6, 2);
    end

== matlab function fec_ber_hw/Soft Demodulation/SSR Soft Demodulation Lane 0/Soft Demodulation 12/symmetric_saturation ==
  data: u input; y output
function y = symmetric_saturation(u)
    if u > 7.75
        y = fi(7.75, 1, 6, 2);
    elseif u < -7.75
        y = fi(-7.75, 1, 6, 2);
    else
        y = fi(u, 1, 6, 2);
    end

== matlab function fec_ber_hw/Encoder/MATLAB Function4 ==
  data: bits input; valid input; frame input size=[160, 1]; tvalid output; lane_0 output size=[1,1]; lane_1 output size=[1,1]; lane_2 output size=[1,1]; lane_3 output; lane_4 output; lane_5 output; lane_6 output; lane_7 output
function [tvalid,lane_0,lane_1,lane_2,lane_3,lane_4,lane_5,lane_6,lane_7] = fcn(bits, valid, frame)

persistent n buffer w buf_i prev_buffer b empty_flag clock_count

if isempty(n)
    n = 160;
    w = 64;
    b = 0;
    prev_buffer = false(1,w*8*4)';
    buffer = false(1,w*8*4)';
    buf_i = 1;
    empty_flag = false;
    lane_0 = uint64(0);
    lane_1 = uint64(0);
    lane_2 = uint64(0);
    lane_3 = uint64(0);
    lane_4 = uint64(0);
    lane_5 = uint64(0);
    lane_6 = uint64(0);
    lane_7 = uint64(0);
    clock_count = 0;
end

clock_count = clock_count + 1;

coder.extrinsic('binaryVectorToDecimal'); 

tvalid = false;
lane_0 = binaryVectorToDecimal(prev_buffer(1:64)','LSBFirst');
lane_1 = binaryVectorToDecimal(prev_buffer(65:128)','LSBFirst');
lane_2 = binaryVectorToDecimal(prev_buffer(129:192)','LSBFirst');
lane_3 = binaryVectorToDecimal(prev_buffer(193:256)','LSBFirst');
lane_4 = binaryVectorToDecimal(prev_buffer(257:320)','LSBFirst');
lane_5 = binaryVectorToDecimal(prev_buffer(321:384)','LSBFirst');
lane_6 = binaryVectorToDecimal(prev_buffer(385:448)','LSBFirst');
lane_7 = binaryVectorToDecimal(prev_buffer(449:512)','LSBFirst');

if valid
    buffer(buf_i:buf_i + n - 1) = frame;
    buf_i = buf_i + n;
    b = b + 160;
end

if ((b >= bits) || (buf_i >= w*8) || empty_flag) && (clock_count > 3)
    empty_flag = false;
    clock_count = 0;
    
    tvalid = true;
    lane_0 = binaryVectorToDecimal(buffer(1:64)','LSBFirst');
    lane_1 = binaryVectorToDecimal(buffer(65:128)','LSBFirst');
    lane_2 = binaryVectorToDecimal(buffer(129:192)','LSBFirst');
    lane_3 = binaryVectorToDecimal(buffer(193:256)','LSBFirst');
    lane_4 = binaryVectorToDecimal(buffer(257:320)','LSBFirst');
    lane_5 = binaryVectorToDecimal(buffer(321:384)','LSBFirst');
    lane_6 = binaryVectorToDecimal(buffer(385:448)','LSBFirst');
    lane_7 = binaryVectorToDecimal(buffer(449:512)','LSBFirst');
    
    prev_buffer = buffer;
    
    temp = buffer(512:buf_i-1);
    buf_i = buf_i - 512;
    buffer = false(1,w*8*4)';
    buffer(1:buf_i) = temp;
    if (b >= bits)
        b = 0;
        if buf_i > 0
            empty_flag = true;
        end
    end
end

== matlab function fec_ber_hw/Soft Demodulation/SSR Soft Demodulation Lane 0/Soft Demodulation 13/symmetric_saturation ==
  data: u input; y output
function y = symmetric_saturation(u)
    if u > 7.75
        y = fi(7.75, 1, 6, 2);
    elseif u < -7.75
        y = fi(-7.75, 1, 6, 2);
    else
        y = fi(u, 1, 6, 2);
    end

== matlab function fec_ber_hw/Soft Demodulation/SSR Soft Demodulation Lane 0/Soft Demodulation 14/symmetric_saturation ==
  data: u input; y output
function y = symmetric_saturation(u)
    if u > 7.75
        y = fi(7.75, 1, 6, 2);
    elseif u < -7.75
        y = fi(-7.75, 1, 6, 2);
    else
        y = fi(u, 1, 6, 2);
    end

== matlab function fec_ber_hw/Soft Demodulation/SSR Soft Demodulation Lane 0/Soft Demodulation 15/symmetric_saturation ==
  data: u input; y output
function y = symmetric_saturation(u)
    if u > 7.75
        y = fi(7.75, 1, 6, 2);
    elseif u < -7.75
        y = fi(-7.75, 1, 6, 2);
    else
        y = fi(u, 1, 6, 2);
    end

== matlab function fec_ber_hw/Soft Demodulation/SSR Soft Demodulation Lane 1/Soft Demodulation 1/symmetric_saturation ==
  data: u input; y output
function y = symmetric_saturation(u)
    if u > 7.75
        y = fi(7.75, 1, 6, 2);
    elseif u < -7.75
        y = fi(-7.75, 1, 6, 2);
    else
        y = fi(u, 1, 6, 2);
    end

== matlab function fec_ber_hw/Soft Demodulation/SSR Soft Demodulation Lane 1/Soft Demodulation 0/symmetric_saturation ==
  data: u input; y output
function y = symmetric_saturation(u)
    if u > 7.75
        y = fi(7.75, 1, 6, 2);
    elseif u < -7.75
        y = fi(-7.75, 1, 6, 2);
    else
        y = fi(u, 1, 6, 2);
    end

== matlab function fec_ber_hw/Soft Demodulation/SSR Soft Demodulation Lane 1/Soft Demodulation 2/symmetric_saturation ==
  data: u input; y output
function y = symmetric_saturation(u)
    if u > 7.75
        y = fi(7.75, 1, 6, 2);
    elseif u < -7.75
        y = fi(-7.75, 1, 6, 2);
    else
        y = fi(u, 1, 6, 2);
    end

== matlab function fec_ber_hw/Soft Demodulation/SSR Soft Demodulation Lane 1/Soft Demodulation 3/symmetric_saturation ==
  data: u input; y output
function y = symmetric_saturation(u)
    if u > 7.75
        y = fi(7.75, 1, 6, 2);
    elseif u < -7.75
        y = fi(-7.75, 1, 6, 2);
    else
        y = fi(u, 1, 6, 2);
    end

== matlab function fec_ber_hw/Soft Demodulation/SSR Soft Demodulation Lane 1/Soft Demodulation 4/symmetric_saturation ==
  data: u input; y output
function y = symmetric_saturation(u)
    if u > 7.75
        y = fi(7.75, 1, 6, 2);
    elseif u < -7.75
        y = fi(-7.75, 1, 6, 2);
    else
        y = fi(u, 1, 6, 2);
    end

== matlab function fec_ber_hw/Soft Demodulation/SSR Soft Demodulation Lane 1/Soft Demodulation 5/symmetric_saturation ==
  data: u input; y output
function y = symmetric_saturation(u)
    if u > 7.75
        y = fi(7.75, 1, 6, 2);
    elseif u < -7.75
        y = fi(-7.75, 1, 6, 2);
    else
        y = fi(u, 1, 6, 2);
    end

== matlab function fec_ber_hw/Soft Demodulation/SSR Soft Demodulation Lane 1/Soft Demodulation 6/symmetric_saturation ==
  data: u input; y output
function y = symmetric_saturation(u)
    if u > 7.75
        y = fi(7.75, 1, 6, 2);
    elseif u < -7.75
        y = fi(-7.75, 1, 6, 2);
    else
        y = fi(u, 1, 6, 2);
    end

== matlab function fec_ber_hw/Soft Demodulation/SSR Soft Demodulation Lane 1/Soft Demodulation 7/symmetric_saturation ==
  data: u input; y output
function y = symmetric_saturation(u)
    if u > 7.75
        y = fi(7.75, 1, 6, 2);
    elseif u < -7.75
        y = fi(-7.75, 1, 6, 2);
    else
        y = fi(u, 1, 6, 2);
    end

== matlab function fec_ber_hw/Soft Demodulation/SSR Soft Demodulation Lane 1/Soft Demodulation 8/symmetric_saturation ==
  data: u input; y output
function y = symmetric_saturation(u)
    if u > 7.75
        y = fi(7.75, 1, 6, 2);
    elseif u < -7.75
        y = fi(-7.75, 1, 6, 2);
    else
        y = fi(u, 1, 6, 2);
    end

== matlab function fec_ber_hw/Soft Demodulation/SSR Soft Demodulation Lane 1/Soft Demodulation 9/symmetric_saturation ==
  data: u input; y output
function y = symmetric_saturation(u)
    if u > 7.75
        y = fi(7.75, 1, 6, 2);
    elseif u < -7.75
        y = fi(-7.75, 1, 6, 2);
    else
        y = fi(u, 1, 6, 2);
    end

== matlab function fec_ber_hw/Soft Demodulation/SSR Soft Demodulation Lane 1/Soft Demodulation 10/symmetric_saturation ==
  data: u input; y output
function y = symmetric_saturation(u)
    if u > 7.75
        y = fi(7.75, 1, 6, 2);
    elseif u < -7.75
        y = fi(-7.75, 1, 6, 2);
    else
        y = fi(u, 1, 6, 2);
    end

== matlab function fec_ber_hw/Soft Demodulation/SSR Soft Demodulation Lane 1/Soft Demodulation 11/symmetric_saturation ==
  data: u input; y output
function y = symmetric_saturation(u)
    if u > 7.75
        y = fi(7.75, 1, 6, 2);
    elseif u < -7.75
        y = fi(-7.75, 1, 6, 2);
    else
        y = fi(u, 1, 6, 2);
    end

== matlab function fec_ber_hw/Soft Demodulation/SSR Soft Demodulation Lane 1/Soft Demodulation 12/symmetric_saturation ==
  data: u input; y output
function y = symmetric_saturation(u)
    if u > 7.75
        y = fi(7.75, 1, 6, 2);
    elseif u < -7.75
        y = fi(-7.75, 1, 6, 2);
    else
        y = fi(u, 1, 6, 2);
    end

== matlab function fec_ber_hw/Soft Demodulation/SSR Soft Demodulation Lane 1/Soft Demodulation 13/symmetric_saturation ==
  data: u input; y output
function y = symmetric_saturation(u)
    if u > 7.75
        y = fi(7.75, 1, 6, 2);
    elseif u < -7.75
        y = fi(-7.75, 1, 6, 2);
    else
        y = fi(u, 1, 6, 2);
    end

== matlab function fec_ber_hw/Soft Demodulation/SSR Soft Demodulation Lane 1/Soft Demodulation 14/symmetric_saturation ==
  data: u input; y output
function y = symmetric_saturation(u)
    if u > 7.75
        y = fi(7.75, 1, 6, 2);
    elseif u < -7.75
        y = fi(-7.75, 1, 6, 2);
    else
        y = fi(u, 1, 6, 2);
    end

== matlab function fec_ber_hw/Soft Demodulation/SSR Soft Demodulation Lane 1/Soft Demodulation 15/symmetric_saturation ==
  data: u input; y output
function y = symmetric_saturation(u)
    if u > 7.75
        y = fi(7.75, 1, 6, 2);
    elseif u < -7.75
        y = fi(-7.75, 1, 6, 2);
    else
        y = fi(u, 1, 6, 2);
    end

== matlab function fec_ber_hw/Encoder/MATLAB Function3 ==
  data: valid_out output; bits input; valid input; lane_0 input; frame_out output size=[80,1] [80..80]; lane_1 input; lane_2 input; lane_3 input; lane_4 input; lane_5 input; lane_6 input; lane_7 input
function [valid_out, frame_out] = fcn(bits, valid, lane_0, lane_1, lane_2, lane_3, lane_4, lane_5, lane_6, lane_7)

persistent frame fixed_frame frame_i fixed_i k w out_flag  bit_count

if isempty(frame)
    k = 80;
    w = 64;
    frame = zeros(1,k)';
    fixed_frame = zeros(1,w*32)';
    frame_i = 1;
    fixed_i = 1;
    out_flag = false;
    bit_count = 0;
end

coder.extrinsic('decimalToBinaryVector'); 

if valid
    fixed_frame(fixed_i:fixed_i+w) = fliplr(decimalToBinaryVector(lane_0,w));
    fixed_i = fixed_i + w;
    fixed_frame(fixed_i:fixed_i+w) = fliplr(decimalToBinaryVector(lane_1,w));
    fixed_i = fixed_i + w;
    fixed_frame(fixed_i:fixed_i+w) = fliplr(decimalToBinaryVector(lane_2,w));
    fixed_i = fixed_i + w;
    fixed_frame(fixed_i:fixed_i+w) = fliplr(decimalToBinaryVector(lane_3,w));
    fixed_i = fixed_i + w;
    fixed_frame(fixed_i:fixed_i+w) = fliplr(decimalToBinaryVector(lane_4,w));
    fixed_i = fixed_i + w;
    fixed_frame(fixed_i:fixed_i+w) = fliplr(decimalToBinaryVector(lane_5,w));
    fixed_i = fixed_i + w;
    fixed_frame(fixed_i:fixed_i+w) = fliplr(decimalToBinaryVector(lane_6,w));
    fixed_i = fixed_i + w;
    fixed_frame(fixed_i:fixed_i+w) = fliplr(decimalToBinaryVector(lane_7,w));
    fixed_i = fixed_i + w;
    out_flag = true;
end

valid_out = out_flag;

if out_flag
    frame = fixed_frame(frame_i:frame_i+(k-1));
    bit_count = bit_count + k;
    frame_i = frame_i + k;
    if (frame_i + k - 1) > fixed_i - 1
        out_flag = false;
        buf = fixed_frame(frame_i:fixed_i - 1);
        fixed_frame = zeros(1,w*32)';
        fixed_i = fixed_i-frame_i;
        frame_i = 1;
        fixed_frame(1:fixed_i) = buf;
        fixed_i = fixed_i + 1;
    end
end

if (bit_count > bits)
    valid_out = false;
end

frame_out = frame(1:80);

== matlab function fec_ber_hw/Decode/MATLAB Function5 ==
  data: bits input; valid input; frame input size=[80, 1]; tvalid output; lane_0 output size=[1,1]; lane_1 output size=[1,1]; lane_2 output size=[1,1]; lane_3 output; lane_4 output; lane_5 output; lane_6 output; lane_7 output
function [tvalid,lane_0,lane_1,lane_2,lane_3,lane_4,lane_5,lane_6,lane_7] = fcn(bits, valid, frame)

persistent k buffer w buf_i prev_buffer

if isempty(k)
    k = 80;
    w = 64;
    prev_buffer = zeros(1,w*8*2)';
    buffer = zeros(1,w*8*2)';
    buf_i = 1;
    lane_0 = uint64(0);
    lane_1 = uint64(0);
    lane_2 = uint64(0);
    lane_3 = uint64(0);
    lane_4 = uint64(0);
    lane_5 = uint64(0);
    lane_6 = uint64(0);
    lane_7 = uint64(0);
end

coder.extrinsic('binaryVectorToDecimal'); 

tvalid = false;
lane_0 = binaryVectorToDecimal(prev_buffer(1:64)','LSBFirst');
lane_1 = binaryVectorToDecimal(prev_buffer(65:128)','LSBFirst');
lane_2 = binaryVectorToDecimal(prev_buffer(129:192)','LSBFirst');
lane_3 = binaryVectorToDecimal(prev_buffer(193:256)','LSBFirst');
lane_4 = binaryVectorToDecimal(prev_buffer(257:320)','LSBFirst');
lane_5 = binaryVectorToDecimal(prev_buffer(321:384)','LSBFirst');
lane_6 = binaryVectorToDecimal(prev_buffer(385:448)','LSBFirst');
lane_7 = binaryVectorToDecimal(prev_buffer(449:512)','LSBFirst');

if valid
    buffer(buf_i:buf_i + k - 1) = frame;
    buf_i = buf_i + k + 1;
end

if buf_i >= bits
    tvalid = true;
    lane_0 = binaryVectorToDecimal(buffer(1:64)','LSBFirst');
    lane_1 = binaryVectorToDecimal(buffer(65:128)','LSBFirst');
    lane_2 = binaryVectorToDecimal(buffer(129:192)','LSBFirst');
    lane_3 = binaryVectorToDecimal(buffer(193:256)','LSBFirst');
    lane_4 = binaryVectorToDecimal(buffer(257:320)','LSBFirst');
    lane_5 = binaryVectorToDecimal(buffer(321:384)','LSBFirst');
    lane_6 = binaryVectorToDecimal(buffer(385:448)','LSBFirst');
    lane_7 = binaryVectorToDecimal(buffer(449:512)','LSBFirst');
    
    prev_buffer = buffer;
    
    temp = buffer(512:buf_i);
    buf_i = buf_i - 512;
    buffer = zeros(1,w*8*2)';
    buffer(1:buf_i) = temp;
end

== matlab function fec_ber_hw/Soft Demodulation/MATLAB Function ==
  data: u input; y output; reset input
function y = max_magnitude(u, reset)
    persistent max
    
    if isempty(max)
        max = fi(0, 0, 32, 24);
    end

   if abs(u) > max
       max(:) = abs(u);
   end
   
   if reset
       max(:) = 0;
   end
   
   y = fi(max, 0, 32, 24);
    
end

== matlab function fec_ber_hw/Soft Demodulation/SSR Soft Demodulation Lane 0/Soft Demodulation 0/symmetric_saturation ==
  data: u input; y output
function y = symmetric_saturation(u)
    if u > 7.75
        y = fi(7.75, 1, 6, 2);
    elseif u < -7.75
        y = fi(-7.75, 1, 6, 2);
    else
        y = fi(u, 1, 6, 2);
    end

== matlab function fec_ber_hw/Soft Demodulation/SSR Soft Demodulation Lane 0/Soft Demodulation 1/symmetric_saturation ==
  data: u input; y output
function y = symmetric_saturation(u)
    if u > 7.75
        y = fi(7.75, 1, 6, 2);
    elseif u < -7.75
        y = fi(-7.75, 1, 6, 2);
    else
        y = fi(u, 1, 6, 2);
    end

== matlab function fec_ber_hw/Decode/MATLAB Function ==
  data: valid input; sample input; frame output size=[160,1] [0..80]; n parameter
function frame = fcn(valid, sample, n)

persistent f count prev_frame

if isempty(f)
    f = zeros(1,160)';
    prev_frame = zeros(1,160)';
    count = 0;
end

frame = prev_frame;

if valid
    count = count + 1;
    f(count) = sample;
end

if count >= n
    prev_frame = f;
    count = 0;
end
